simulink model "pr4-PD"  (R2019b)
settings: Solver=VariableStepAuto  StartTime=0.0  StopTime=100  RelTol=1e-3
libraries: fuzblock x1
settings Model: Creator=pablo  LastModifiedBy=pablo

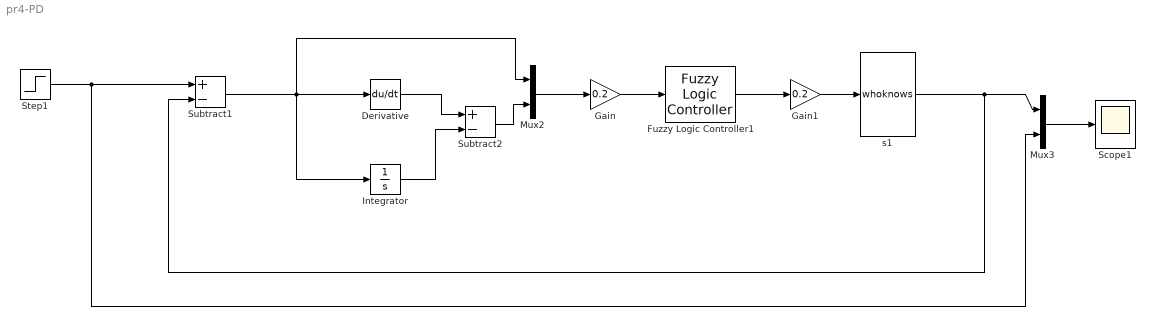
== system pr4-PD ==
  Derivative : Derivative
  Fuzzy Logic Controller1 : fuzblock/Fuzzy Logic  Controller  FIS='prueba.fis'  OutputSampleNumber=101  DataType=double  FuzzifiedInputs=off  RuleFiringStrengths=off  RuleOutputs=off  AggregatedOutputs=off  SimulateUsing=Interpreted execution  OutOfRangeInputValueMessage=warning  NoRuleFiredMessage=warning  EmptyOutputFuzzySetMessage=warning
  Gain : Gain  Gain=0.2
  Gain1 : Gain  Gain=0.2
  Integrator : Integrator
  Mux2 : Mux  Inputs=2
  Mux3 : Mux  Inputs=2
  Scope1 : Scope
  Step1 : Step  SampleTime=0
  Subtract1 : Sum  Inputs=+-
  Subtract2 : Sum  Inputs=+-
  s1 : M-S-Function  FunctionName=whoknows  Parameters=L, P1, P2, T, R  mask{L=7, P1=0, P2=7, T=1, R=0}
      mask prompts: L "Laboratorio"; P1 "Primer digito del Puesto"; P2 "Segundo digito del Puesto"; T "Tipo de Planta"; R "Ruido"
      mask Display: disp('Sistema')
  wires:
  Step1/1 -> Mux3/2, Subtract1/1
  Mux3/1 -> Scope1/1
  s1/1 -> Mux3/1, Subtract1/2
  Subtract1/1 -> Derivative/1, Integrator/1, Mux2/1
  Mux2/1 -> Gain/1
  Fuzzy Logic Controller1/1 -> Gain1/1
  Integrator/1 -> Subtract2/2
  Derivative/1 -> Subtract2/1
  Subtract2/1 -> Mux2/2
  Gain/1 -> Fuzzy Logic Controller1/1
  Gain1/1 -> s1/1
